simulink model "model_1"  (R2021b)
settings: Solver=VariableStepAuto  StartTime=0.0  StopTime=5  RelTol=1e-3
values from neighbouring files (symbols this model uses):
  A1 = [10, 7, 8; 2, 15, 10; 3, 11, 12]    [task_1.m]    (also in task_3.m = [1, 1, 0; -1, 1, 0; 0, 0, -3]; task_4.m = [1, 1, 0; -1, 1, 0; 0, 0, -3]; task_5.m = [0 1; 0 0]; untitled2.m = [-3 0 0; 0 4 2; 0 -2 4])
  A2 = [0.5, 2, 0, 0; -2, 0.5, 0, 0; 0, 0, 0.3, 1; 0, 0, -1, 0.3]    [task_1.m]    (also in task_3.m = [0 5 0; -5 0 0; 0 0 0.01]; task_4.m = [0 5 0; -5 0 0; 0 0 0.01]; task_5.m = [0 1 0 0 0 0; -1 0 0 0 0 0; 0 0 0 3 0 0; 0 0 -3 0 0 0; untitled2.m = [0 5 0 0; -5 0 0 0; 0 0 0 2; 0 0 -2 0])
  B1 = [1;2;3]    [task_1.m]    (also in task_3.m = [1;1;1]; task_4.m = [1;1;1]; task_5.m = [0; 1]; untitled2.m = [1; 1; 1])
  B2 = [1, 1, 1, 1; 1, 2, 3, 4; 1, 2, 3, 4]    [task_1.m]    (also in task_3.m = [1,1,1;1,1,1;1,1,1]; task_4.m = [1,1,1;1,1,1;1,1,1]; task_5.m = [0 0 0 0 0 0; 0 0 0 0 0 0]; untitled2.m = [1 0 0 0; 0 1 0 0; 0 0 1 1])
  C2 = [1, 1, 1]    [task_1.m]    (also in task_3.m; task_4.m; task_5.m = -C1; untitled2.m = [1 1 1])
  D2 = zeros(1, 4)    [task_1.m]    (also in task_3.m = [-1, -1, -1]; task_4.m = [-1, -1, -1]; task_5.m = [8/pi 0 8/(3*pi) 0 8/(5*pi) 0]; untitled2.m = [-1 -1 -1 -1])
  K1 = -Y1*inv(P1)    [task_1.m]    (also in task_3.m; task_4.m; task_5.m = -y*inv(p); untitled2.m = -y*inv(p))
  K2 = Y2 - K1*P2    [task_1.m]    (also in task_3.m; task_4.m; task_5.m = Y - K1*P; untitled2.m = Y - K1*P)
settings Model: Creator=vital  LastModifiedBy=vital

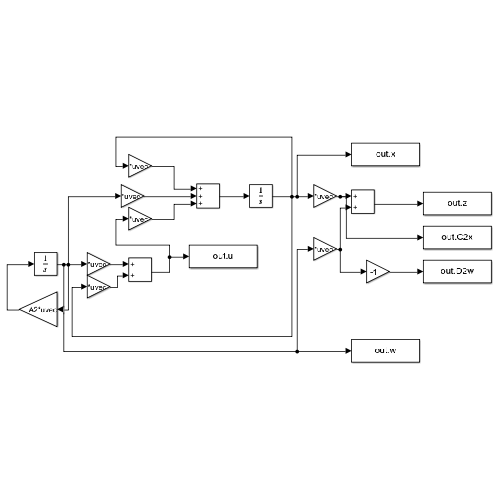
[thumbnail: Simulink's stored preview of the top-level diagram]
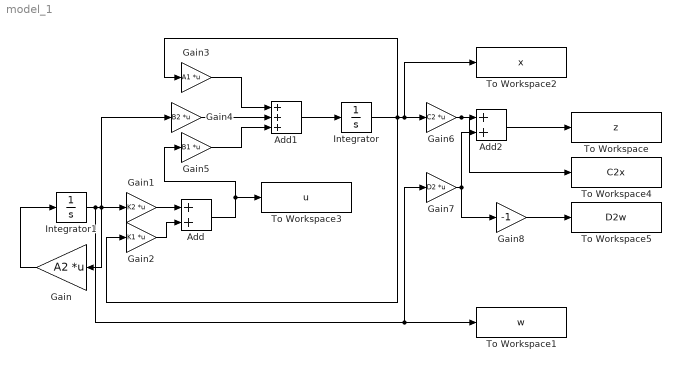
== system model_1 ==
  Add : Sum
  Add1 : Sum  Inputs=+++
  Add2 : Sum
  Gain : Gain  Gain=A2  Multiplication=Matrix(K*u) (u vector)
  Gain1 : Gain  Gain=K2  Multiplication=Matrix(K*u) (u vector)
  Gain2 : Gain  Gain=K1  Multiplication=Matrix(K*u) (u vector)
  Gain3 : Gain  Gain=A1  Multiplication=Matrix(K*u) (u vector)
  Gain4 : Gain  Gain=B2  Multiplication=Matrix(K*u) (u vector)
  Gain5 : Gain  Gain=B1  Multiplication=Matrix(K*u) (u vector)
  Gain6 : Gain  Gain=C2  Multiplication=Matrix(K*u) (u vector)
  Gain7 : Gain  Gain=D2  Multiplication=Matrix(K*u) (u vector)
  Gain8 : Gain  Gain=-1
  Integrator : Integrator
  Integrator1 : Integrator  InitialCondition=[1;1;1;1]
  To Workspace : ToWorkspace  VariableName=z  SaveFormat=Timeseries  SampleTime=-1
  To Workspace1 : ToWorkspace  VariableName=w  SaveFormat=Timeseries  SampleTime=-1
  To Workspace2 : ToWorkspace  VariableName=x  SaveFormat=Timeseries  SampleTime=0.0001
  To Workspace3 : ToWorkspace  VariableName=u  SaveFormat=Timeseries  SampleTime=-1
  To Workspace4 : ToWorkspace  VariableName=C2x  SaveFormat=Timeseries  SampleTime=-1
  To Workspace5 : ToWorkspace  VariableName=D2w  SaveFormat=Timeseries  SampleTime=-1
  wires:
  Integrator1/1 -> Gain4/1, Gain1/1, Gain/1, Gain7/1, To Workspace1/1
  Gain2/1 -> Add/2
  Gain1/1 -> Add/1
  Integrator/1 -> To Workspace2/1, Gain6/1, Gain3/1, Gain2/1
  Gain4/1 -> Add1/2
  Gain3/1 -> Add1/1
  Add/1 -> To Workspace3/1, Gain5/1
  Gain5/1 -> Add1/3
  Add1/1 -> Integrator/1
  Gain/1 -> Integrator1/1
  Gain7/1 -> Add2/2, Gain8/1
  Add2/1 -> To Workspace/1
  Gain6/1 -> To Workspace4/1, Add2/1
  Gain8/1 -> To Workspace5/1
